simulink library "Quat2Rot"  (R2014b)
settings: Solver=ode45  StartTime=0.0  StopTime=10.0  RelTol=1e-3
settings Model: Creator=Hp  LastModifiedBy=Hp

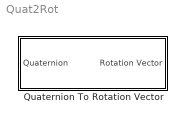
== system Quat2Rot ==
  Quaternion To Rotation Vector : Subsystem

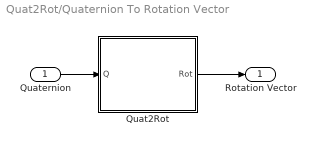
== system Quat2Rot/Quaternion To Rotation Vector ==
  Quaternion : Inport
  Quat2Rot : MATLAB Function  TreatAsAtomicUnit=on
  Rotation Vector : Outport
  wires:
  Quaternion/1 -> Quat2Rot/1(Q)
  Quat2Rot/1(Rot) -> Rotation Vector/1

== matlab function Quat2Rot/Quaternion To Rotation Vector/Quat2Rot ==
  data: Q input; Rot output
function Rot=Quat2Rot(Q)
% Returns a vector whose norm corresponds to the rotation angle
% (between 0 and pi) of quaternion Q
if norm(Q)==0
    Rot=[0;0;0];
else
    Q=Q/norm(Q);
    if Q(1)<0
        Q=-Q; % Positive real part
    end   
    w=Q(1);q=Q(2:4);
    if w==1
        Rot=[0;0;0];
    else
        Rot=2*atan2(norm(q),w)*q/norm(q);  % Euler vector
    end
end
end
